simulink model "Cruise_Model_V16"  (R2024a)
settings: Solver=ode23t  StartTime=0.0  StopTime=t5(end)  RelTol=1e-3
values from neighbouring files (symbols this model uses):
  coefficients =     [UAM2.mat]    (also in VX4_cur.mat; VX4data.mat; alexisignoringme11UAM2.mat; alexisignoringme12.mat)
  idxf = [1 78 155 231 308 385 462 538 615 692 769 845 ... (70 elements, 1x70)]    [alexisignoringme.mat]    (also in alexisignoringme11UAM2.mat = [1 112 223 334 445 555 666 777 888 999 1001 1112 ... (50 ele; alexisignoringme12.mat = [1 54 106 159 211 264 316 369 421 474 526 579 ... (100 eleme; alexisignoringme13.mat = [1 54 106 159 211 264 316 369 421 474 526 579 ... (100 eleme; alexisignoringme14.mat = [1 500 999 1001 1500 1999 2001 2500 2999 3001 3500 3999 ... )
  Kpi = lqr(sys, Q, R)    [QRerr_LQI.m]    (also in alexisignoringme8.mat = [9.62344892608e-17 -1.21933000029e-16 1.4312558077e-15 29.45)
  missionruntime =     [alexisignoringme4.mat]    (also in alexisignoringme5.mat; alexisignoringme6.mat; alexisignoringme7.mat; alexisignoringme8.mat)
  q = 0.5*1.225*airflow.U^2    [VLMV3.m]    (also in VLMV3_modified.m = 0.5*1.225*airflow.U^2*Sref)
  Ut = [0 0 -4.89661324026e-08 0 0 -1504.57476188 -0.000428335964898 -1.57410795509e-09 3.42121377805e-06 0 0 0 ... (450 elements, 9x50)]    [alexisignoringme5.mat]    (also in alexisignoringme6.mat; alexisignoringme7.mat; alexisignoringme8.mat = [0 0 0 0 0 -1498.96331992 -4.41873387445e-05 -1.31180695462e)
  uvec = [0.1 3.42222222222 6.74444444444 10.0666666667 13.3888888889 16.7111111111 20.0333333333 23.3555555556 26.6777777778 30]    [alexisignoringme.mat]    (also in alexisignoringme4.mat; alexisignoringme5.mat; alexisignoringme6.mat; alexisignoringme7.mat)
  X = [0.00351660116596 0 -9.99999602467 0 0 0 2.75026701025e-08 -4.1982332666e-06 -1.5333765693e-08 0.000503097278932 0 -6.54626389426e-11 ... (630 elements, 9x5x14)]    [alexisignoringme.mat]    (also in alexisignoringme12.mat = [0.000256495736971 0 -9.99999647184 0 0 0 0 -3.73764411116e-; alexisignoringme13.mat = [0.00833666803911 0 -10.0000021435 0 0 0 0 7.14203458163e-06; alexisignoringme14.mat = [0.00833666803911 0 -10.0000021435 0 0 0 0 7.14203458163e-06; alexisignoringme4.mat = [0.00351658839646 0 -9.99999599468 0 0 0 2.7327442949e-09 -4)
  Xes = X(:,idx(4))    [QRerr_LQI.m]    (also in QRerr_p.m = X(:,idx(2)); alexisignoringme4.mat = [0.00351658839646 0 -9.99999599468 0 0 0 2.7327442949e-09 -4; alexisignoringme5.mat = [0 0 -1.11199998303 0 0 0 -1.38069247376e-09 1.48137256273e-; alexisignoringme6.mat = [0 0 -1.11199998303 0 0 0 -1.38069247376e-09 1.48137256273e-)
undefined symbols (not defined in the file or in its folder): F, Light, MIL, tl, VX4, xvec
libraries: slpidlib x14, aerolibwind2 x8, aerolibatmos2 x4, shared6dof x1
(part 2 of 3)

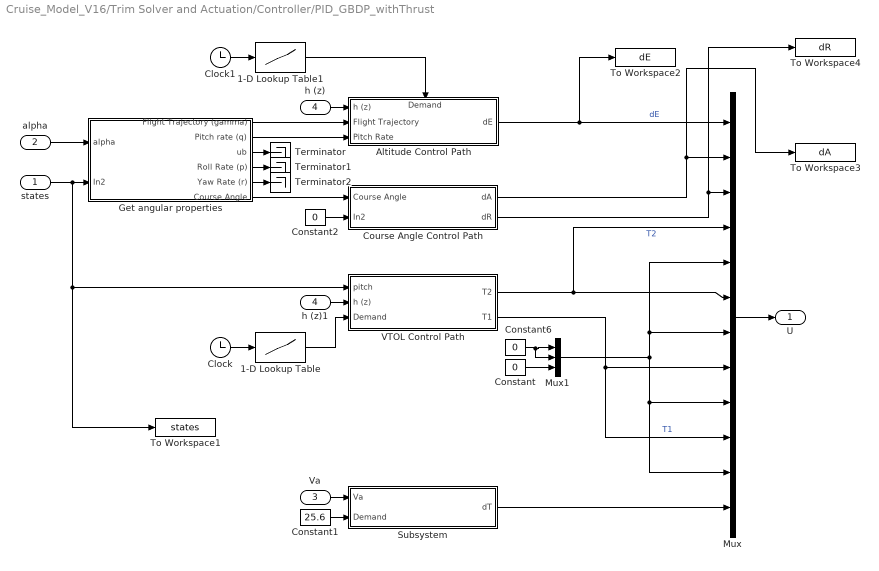
== system Cruise_Model_V16/Trim Solver and Actuation/Controller/PID_GBDP_withThrust ==
  states : Inport
  alpha : Inport  Port=2
  Va : Inport  Port=3
  h (z) : Inport  Port=4
  1-D Lookup Table : Lookup_n-D  NumberOfTableDimensions=1  BreakpointsForDimension1=[mission.trans.t mission.cruise.t(2:end)]  Table=[mission.trans.altitude 0*ones(size(mission.trans.altitude(2:end)))]  InternalRulePriority=Speed  RndMeth=Simplest
  1-D Lookup Table1 : Lookup_n-D  NumberOfTableDimensions=1  BreakpointsForDimension1=[mission.trans.t mission.cruise.t(2:end)]  Table=[mission.trans.altitude mission.cruise.altitude(2:end)]  InternalRulePriority=Speed  RndMeth=Simplest
  Altitude Control Path : Subsystem
      settings: PortSchema="{\"entries\":[{\"content\":{\"sides\":[{\"content\":{\"connectorIds\":[\"In1\",\"In2\",\"In3\"]},\"type\":\"ConnectorPlacement.EquallySpacedRectSide\",\"uuid\":\"675ebe7b-8fa8-41fa-ad50-d7fa74657396\"},{\"content\":{\"connectorIds\":[\"Out1\"],\"side\":\"RIGHT\"},\"type\":\"ConnectorPlacement.EquallySpacedRectSide\",\"uuid\":\"13b074cf-565d-449c-ab17-946bdb38993a\"},{\"content\":{\"connectorIds\":[\"In4\"],\"side\":\"TOP\"},\"type\":\"ConnectorPlacement.EquallySpacedRectSide\",\"uuid\":\"a25968b9-1287-4975-9ac3-b2da8f663380\"}]},\"type\":\"ConnectorPlacement.EquallySpacedConnector\",\"uuid\":\"28fe7750-cc88-4371-bcf6-f4778a62f5aa\"}],\"packageUris\":[\"http://schema.mathworks.com/mf0/Connector/R2020b\"],\"version\":\"1.0\"}"
  Clock : Clock
  Clock1 : Clock
  Constant : Constant  Value=0
  Constant1 : Constant  Value=25.6
  Constant2 : Constant  Value=0
  Constant6 : Constant  Value=0
  Course Angle Control Path : Subsystem
  Get angular properties : Subsystem
  Mux : Mux  Inputs=12
  Mux1 : Mux  Inputs=3
  Subsystem : Subsystem
  Terminator : Terminator
  Terminator1 : Terminator
  Terminator2 : Terminator
  To Workspace1 : ToWorkspace  VariableName=states  SaveFormat=Timeseries  SampleTime=-1
  To Workspace2 : ToWorkspace  VariableName=dE  SaveFormat=Timeseries  SampleTime=-1
  To Workspace3 : ToWorkspace  VariableName=dA  SaveFormat=Timeseries  SampleTime=-1
  To Workspace4 : ToWorkspace  VariableName=dR  SaveFormat=Timeseries  SampleTime=-1
  VTOL Control Path : Subsystem
  h (z)1 : InportShadow  Port=4
  U : Outport
  wires:
  Mux/1 -> U/1
  Get angular properties/5(Yaw Rate (r)) -> Terminator2/1
  Get angular properties/4(Roll Rate (p)) -> Terminator1/1
  alpha/1 -> Get angular properties/1(alpha)
  Get angular properties/3(ub) -> Terminator/1
  states/1 -> To Workspace1/1, VTOL Control Path/1(pitch), Get angular properties/2(In2)
  Mux1/1 -> Mux/5, Mux/7, Mux/11, Mux/9
  Constant6/1 -> Mux1/1, Mux1/2
  Constant/1 -> Mux1/3
  h (z)/1 -> Altitude Control Path/1(h (z))
  1-D Lookup Table1/1 -> Altitude Control Path/4(Demand)
  Get angular properties/1(Flight Trajectory (gamma)) -> Altitude Control Path/2(Flight Trajectory)
  Get angular properties/2(Pitch rate (q)) -> Altitude Control Path/3(Pitch Rate)
  Get angular properties/6(Course Angle) -> Course Angle Control Path/1(Course Angle)
  Va/1 -> Subsystem/1(Va)
  Constant1/1 -> Subsystem/2(Demand)
  Altitude Control Path/1(dE) -> Mux/1, To Workspace2/1  "dE"
  Course Angle Control Path/1(dA) -> To Workspace3/1, Mux/2
  Course Angle Control Path/2(dR) -> To Workspace4/1, Mux/3
  Clock/1 -> 1-D Lookup Table/1
  1-D Lookup Table/1 -> VTOL Control Path/3(Demand)
  h (z)1/1 -> VTOL Control Path/2(h (z))
  Clock1/1 -> 1-D Lookup Table1/1
  VTOL Control Path/1(T2) -> Mux/4, Mux/6  "T2"
  VTOL Control Path/2(T1) -> Mux/10, Mux/8  "T1"
  Subsystem/1(dT) -> Mux/12
  Constant2/1 -> Course Angle Control Path/2(In2)

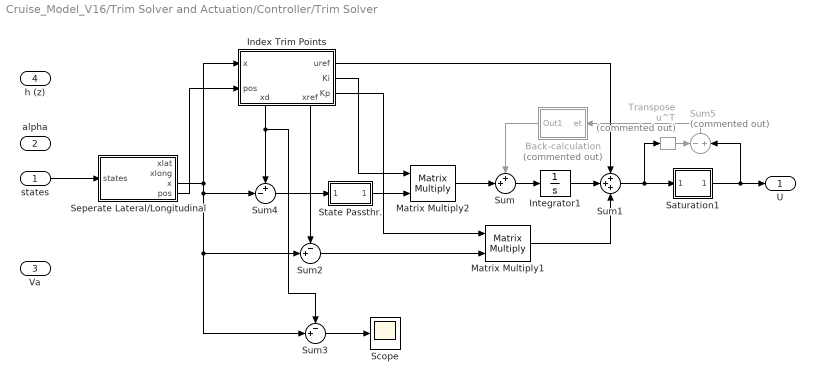
== system Cruise_Model_V16/Trim Solver and Actuation/Controller/Trim Solver ==
  states : Inport
  alpha : Inport  Port=2
  Va : Inport  Port=3
  h (z) : Inport  Port=4
  Back-calculation : Subsystem  Commented=on
  Index Trim Points : Subsystem
      settings: PortSchema="{\"entries\":[{\"content\":{\"sides\":[{\"content\":{\"connectorIds\":[\"In1\",\"In2\"]},\"type\":\"ConnectorPlacement.EquallySpacedRectSide\",\"uuid\":\"3e759be8-b0b5-4bdb-bb26-96e56af52772\"},{\"content\":{\"connectorIds\":[\"Out1\",\"Out2\",\"Out3\"],\"side\":\"RIGHT\"},\"type\":\"ConnectorPlacement.EquallySpacedRectSide\",\"uuid\":\"8308db73-24aa-4a70-a5f0-9ec5de8c120a\"},{\"content\":{\"side\":\"TOP\"},\"type\":\"ConnectorPlacement.EquallySpacedRectSide\",\"uuid\":\"2166a8af-7157-44fc-b4c0-6126f30836aa\"},{\"content\":{\"connectorIds\":[\"Out4\",\"Out5\"],\"side\":\"BOTTOM\"},\"type\":\"ConnectorPlacement.EquallySpacedRectSide\",\"uuid\":\"144aeecd-f2ed-4e8c-a5f9-9bd63c6f3635\"}]},\"type\":\"ConnectorPlacement.EquallySpacedConnector\",\"uuid\":\"70cf00ba-20c2-419b-abed-4793342c0662\"}],\"packageUris\":[\"http://schema.mathworks.com/mf0/Connector/R2020b\"],\"version\":\"1.0\"}"
  Integrator1 : Integrator
  Matrix Multiply1 : Product  Multiplication=Matrix(*)
  Matrix Multiply2 : Product  Multiplication=Matrix(*)
  Saturation1 : Subsystem
  Scope : Scope
  Seperate Lateral/Longitudinal : Subsystem
  State Passthr. : Subsystem
  Sum : Sum  Inputs=++|
  Sum1 : Sum  Inputs=+++
  Sum2 : Sum  Inputs=-+|
  Sum3 : Sum  Inputs=-+|
  Sum4 : Sum  Inputs=+-|
  Sum5 : Sum  Commented=on  Inputs=-|+
  Transpose : Math  Commented=on  Operator=transpose
  U : Outport
  wires:
  states/1 -> Seperate Lateral/Longitudinal/1(states)
  Index Trim Points/1(uref) -> Sum1/1
  Index Trim Points/4(xd) -> Sum3/1, Sum4/1
  Seperate Lateral/Longitudinal/3(x) -> Sum2/2, Sum3/2, Sum4/2, Index Trim Points/1(x)
  Index Trim Points/5(xref) -> Sum2/1
  Index Trim Points/3(Kp) -> Matrix Multiply1/1
  Index Trim Points/2(Ki) -> Matrix Multiply2/1
  Sum4/1 -> State Passthr./1(In2)
  State Passthr./1(Out4) -> Matrix Multiply2/2
  Sum2/1 -> Matrix Multiply1/2
  Sum1/1 -> Saturation1/1(In1), Transpose/1
  Matrix Multiply2/1 -> Sum/2
  Sum/1 -> Integrator1/1
  Transpose/1 -> Sum5/1
  Sum5/1 -> Back-calculation/1(et)
  Integrator1/1 -> Sum1/2
  Matrix Multiply1/1 -> Sum1/3
  Back-calculation/1(Out1) -> Sum/1
  Sum3/1 -> Scope/1
  Saturation1/1(Out1) -> Sum5/2, U/1
  Seperate Lateral/Longitudinal/4(pos) -> Index Trim Points/2(pos)

== system Cruise_Model_V16/Atmospheric Effects/Atmospheric Effects1/Variant Subsystem/a ==
  h (z) : Inport
  Constant : Constant  Value=0
  ISA Atmosphere : aerolibatmos2/ISA Atmosphere Model  useExtended=off  action=Warning  custom=off  viscosityOut=off  g=9.80665  gamma=1.4  R=287.0531  L=0.0065  h_trop=11000  h_strat=20000  rho0=1.225  P0=101325  T0=288.15  h0=0  S=110.4  Tref=273.15  muref=1.716e-5
  Terminator1 : Terminator
  Terminator2 : Terminator
  Terminator3 : Terminator
  Air Density : Outport
  Vw : Outport  Port=2
  wires:
  h (z)/1 -> ISA Atmosphere/1
  ISA Atmosphere/2 -> Terminator1/1
  ISA Atmosphere/1 -> Terminator3/1
  ISA Atmosphere/4 -> Air Density/1
  ISA Atmosphere/3 -> Terminator2/1
  Constant/1 -> Vw/1

== system Cruise_Model_V16/Atmospheric Effects/Atmospheric Effects1/Variant Subsystem/ag ==
  uvw_e : Inport
  h (z) : Inport  Port=2
  Demux : Demux  Outputs=3
  Discrete Wind Gust Model : aerolibwind2/Discrete Wind Gust Model  units=Metric (MKS)  Gx=on  Gy=on  Gz=on  t_0=40  d_m=[120 120 80]  v_m=[10 10 10]
  ISA Atmosphere : aerolibatmos2/ISA Atmosphere Model  custom=off  g=9.80665  gamma=1.4  R=287.0531  L=0.0065  h_trop=11000  h_strat=20000  rho0=1.225  P0=101325  T0=288.15  h0=0
  Terminator1 : Terminator
  Terminator2 : Terminator
  Terminator3 : Terminator
  Vw : Outport
  Air Density : Outport  Port=2
  wires:
  h (z)/1 -> ISA Atmosphere/1
  Demux/1 -> Discrete Wind Gust Model/1
  ISA Atmosphere/2 -> Terminator1/1
  ISA Atmosphere/1 -> Terminator3/1
  ISA Atmosphere/4 -> Air Density/1
  uvw_e/1 -> Demux/1
  ISA Atmosphere/3 -> Terminator2/1
  Discrete Wind Gust Model/1 -> Vw/1

== system Cruise_Model_V16/Atmospheric Effects/Atmospheric Effects1/Variant Subsystem/agt ==
  <uvw_e> : Inport
  DCM : Inport  Port=2
  h (z) : Inport  Port=3
  Demux : Demux  Outputs=3
  Discrete Wind Gust Model : aerolibwind2/Discrete Wind Gust Model  units=Metric (MKS)  Gx=on  Gy=on  Gz=on  t_0=40  d_m=[120 120 80]  v_m=[10 10 10]
  Dryden Wind Turbulence Model (Discrete (+q +r)) : aerolibwind2/Dryden Wind Turbulence Model  (Continuous (+q -r))  units=Metric (MKS)  spec=MIL-F-8785C  model=Continuous Dryden (+q -r)  W20=10  Wdeg=8  TurbProb=10^-2 - Light  L_high=533.4  Wingspan=7  ts=0.1  Seed=[23341 23342 23343 23344]  T_on=on
      settings: LibrarySourceBlock=|
      | aerolibwind2/Dryden Wind Turbulence Model
      | (Discrete (+q +r))
  ISA Atmosphere : aerolibatmos2/ISA Atmosphere Model  custom=off  g=9.80665  gamma=1.4  R=287.0531  L=0.0065  h_trop=11000  h_strat=20000  rho0=1.225  P0=101325  T0=288.15  h0=0
  Sum : Sum  Inputs=|++
  Terminator{,1..3} (4 alike) : Terminator
  Vw : Outport
  Air Density : Outport  Port=2
  wires:
  h (z)/1 -> Dryden Wind Turbulence Model (Discrete (+q +r))/1, ISA Atmosphere/1
  Demux/1 -> Dryden Wind Turbulence Model (Discrete (+q +r))/2, Discrete Wind Gust Model/1
  ISA Atmosphere/2 -> Terminator1/1
  ISA Atmosphere/1 -> Terminator3/1
  ISA Atmosphere/4 -> Air Density/1
  <uvw_e>/1 -> Demux/1
  DCM/1 -> Dryden Wind Turbulence Model (Discrete (+q +r))/3
  Dryden Wind Turbulence Model (Discrete (+q +r))/2 -> Terminator/1
  Sum/1 -> Vw/1
  ISA Atmosphere/3 -> Terminator2/1
  Dryden Wind Turbulence Model (Discrete (+q +r))/1 -> Sum/2
  Discrete Wind Gust Model/1 -> Sum/1

== system Cruise_Model_V16/Atmospheric Effects/Atmospheric Effects1/Variant Subsystem/at ==
  uvw_e : Inport
  DCM : Inport  Port=2
  h (z) : Inport  Port=3
  Demux : Demux  Outputs=3
  Dryden Wind Turbulence Model (Discrete (+q +r)) : aerolibwind2/Dryden Wind Turbulence Model  (Continuous (+q -r))  units=Metric (MKS)  spec=MIL-F-8785C  model=Continuous Dryden (+q -r)  W20=10  Wdeg=8  TurbProb=10^-2 - Light  L_high=533.4  Wingspan=7  ts=0.1  Seed=[23341 23342 23343 23344]  T_on=on
      settings: LibrarySourceBlock=|
      | aerolibwind2/Dryden Wind Turbulence Model
      | (Discrete (+q +r))
  ISA Atmosphere : aerolibatmos2/ISA Atmosphere Model  custom=off  g=9.80665  gamma=1.4  R=287.0531  L=0.0065  h_trop=11000  h_strat=20000  rho0=1.225  P0=101325  T0=288.15  h0=0
  Terminator{,1..5} (6 alike) : Terminator
  Vw : Outport
  Air Density : Outport  Port=2
  wires:
  h (z)/1 -> Dryden Wind Turbulence Model (Discrete (+q +r))/1, ISA Atmosphere/1
  Demux/1 -> Dryden Wind Turbulence Model (Discrete (+q +r))/2
  ISA Atmosphere/2 -> Terminator1/1
  ISA Atmosphere/1 -> Terminator3/1
  ISA Atmosphere/4 -> Air Density/1
  uvw_e/1 -> Demux/1
  DCM/1 -> Dryden Wind Turbulence Model (Discrete (+q +r))/3
  Dryden Wind Turbulence Model (Discrete (+q +r))/2 -> Terminator/1
  ISA Atmosphere/3 -> Terminator2/1
  Demux/2 -> Terminator4/1
  Demux/3 -> Terminator5/1
  Dryden Wind Turbulence Model (Discrete (+q +r))/1 -> Vw/1

== system Cruise_Model_V16/Atmospheric Effects/Atmospheric Effects1/Variant Subsystem/g ==
  uvw_e : Inport
  Constant : Constant  Value=1.225
  Demux : Demux  Outputs=3
  Discrete Wind Gust Model : aerolibwind2/Discrete Wind Gust Model  units=Metric (MKS)  Gx=on  Gy=on  Gz=on  t_0=40  d_m=[120 120 80]  v_m=[10 10 10]
  Vw : Outport
  Air Density : Outport  Port=2
  wires:
  Demux/1 -> Discrete Wind Gust Model/1
  uvw_e/1 -> Demux/1
  Discrete Wind Gust Model/1 -> Vw/1
  Constant/1 -> Air Density/1

== system Cruise_Model_V16/Atmospheric Effects/Atmospheric Effects1/Variant Subsystem/gt ==
  <uvw_e> : Inport
  DCM : Inport  Port=2
  h (z) : Inport  Port=3
  Constant : Constant  Value=1.225
  Demux : Demux  Outputs=3
  Discrete Wind Gust Model : aerolibwind2/Discrete Wind Gust Model  units=Metric (MKS)  Gx=on  Gy=on  Gz=on  t_0=40  d_m=[120 120 80]  v_m=[10 10 10]
  Dryden Wind Turbulence Model (Discrete (+q +r)) : aerolibwind2/Dryden Wind Turbulence Model  (Continuous (+q -r))  units=Metric (MKS)  spec=MIL-F-8785C  model=Continuous Dryden (+q -r)  W20=10  Wdeg=8  TurbProb=10^-2 - Light  L_high=533.4  Wingspan=7  ts=0.1  Seed=[23341 23342 23343 23344]  T_on=on
      settings: LibrarySourceBlock=|
      | aerolibwind2/Dryden Wind Turbulence Model
      | (Discrete (+q +r))
  Sum : Sum  Inputs=|++
  Terminator : Terminator
  Vw : Outport
  Air Density : Outport  Port=2
  wires:
  h (z)/1 -> Dryden Wind Turbulence Model (Discrete (+q +r))/1
  Demux/1 -> Dryden Wind Turbulence Model (Discrete (+q +r))/2, Discrete Wind Gust Model/1
  <uvw_e>/1 -> Demux/1
  DCM/1 -> Dryden Wind Turbulence Model (Discrete (+q +r))/3
  Dryden Wind Turbulence Model (Discrete (+q +r))/2 -> Terminator/1
  Sum/1 -> Vw/1
  Dryden Wind Turbulence Model (Discrete (+q +r))/1 -> Sum/2
  Discrete Wind Gust Model/1 -> Sum/1
  Constant/1 -> Air Density/1

== system Cruise_Model_V16/Atmospheric Effects/Atmospheric Effects1/Variant Subsystem/n ==
  Constant : Constant  Value=0
  Constant1 : Constant  Value=1.225
  Vw : Outport
  Air Density : Outport  Port=2
  wires:
  Constant/1 -> Vw/1
  Constant1/1 -> Air Density/1

== system Cruise_Model_V16/Atmospheric Effects/Atmospheric Effects1/Variant Subsystem/t ==
  <uvw_e> : Inport
  DCM : Inport  Port=2
  h (z) : Inport  Port=3
  Constant1 : Constant  Value=1.225
  Demux : Demux  Outputs=3
  Dryden Wind Turbulence Model (Discrete (+q +r)) : aerolibwind2/Dryden Wind Turbulence Model  (Continuous (+q -r))  units=Metric (MKS)  spec=MIL-F-8785C  model=Continuous Dryden (+q -r)  W20=10  Wdeg=8  TurbProb=10^-2 - Light  L_high=533.4  Wingspan=7  ts=0.1  Seed=[23341 23342 23343 23344]  T_on=on
      settings: LibrarySourceBlock=|
      | aerolibwind2/Dryden Wind Turbulence Model
      | (Discrete (+q +r))
  Terminator : Terminator
  Vw : Outport
  Air Density : Outport  Port=2
  wires:
  h (z)/1 -> Dryden Wind Turbulence Model (Discrete (+q +r))/1
  Demux/1 -> Dryden Wind Turbulence Model (Discrete (+q +r))/2
  <uvw_e>/1 -> Demux/1
  DCM/1 -> Dryden Wind Turbulence Model (Discrete (+q +r))/3
  Dryden Wind Turbulence Model (Discrete (+q +r))/2 -> Terminator/1
  Constant1/1 -> Air Density/1
  Dryden Wind Turbulence Model (Discrete (+q +r))/1 -> Vw/1

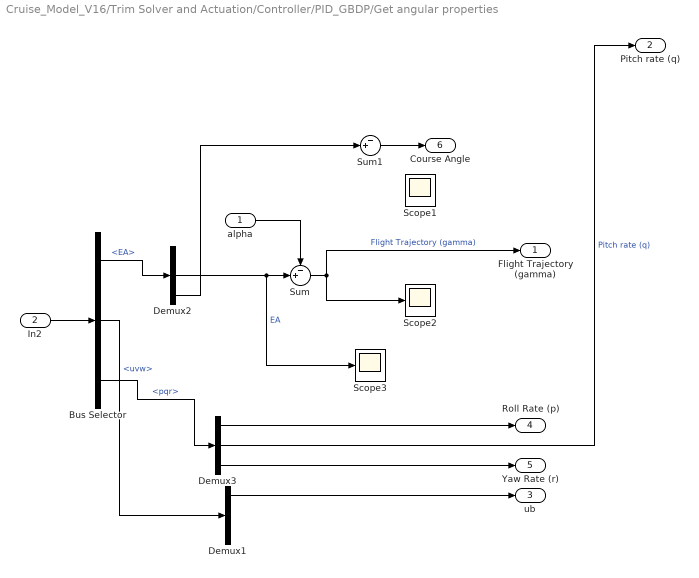
== system Cruise_Model_V16/Trim Solver and Actuation/Controller/PID_GBDP/Get angular properties ==
  alpha : Inport
  In2 : Inport  Port=2
  Bus Selector : BusSelector  OutputSignals=EA,uvw,pqr
  Demux1 : Demux  Outputs=3
  Demux2 : Demux  Outputs=3
  Demux3 : Demux  Outputs=3
  Scope1 : Scope
  Scope2 : Scope
  Scope3 : Scope
  Sum : Sum  Inputs=-+|
  Sum1 : Sum  Inputs=-+|
  Flight Trajectory (gamma) : Outport
  Pitch rate (q) : Outport  Port=2
  ub : Outport  Port=3
  Roll Rate (p) : Outport  Port=4
  Yaw Rate (r) : Outport  Port=5
  Course Angle : Outport  Port=6
  wires:
  alpha/1 -> Sum/1
  Demux2/2 -> Sum/2, Scope3/1  "EA"
  Bus Selector/3 -> Demux3/1  "<pqr>"
  Sum/1 -> Flight Trajectory (gamma)/1, Scope2/1  "Flight Trajectory (gamma)"
  Bus Selector/1 -> Demux2/1  "<EA>"
  In2/1 -> Bus Selector/1
  Demux3/2 -> Pitch rate (q)/1  "Pitch rate (q)"
  Bus Selector/2 -> Demux1/1  "<uvw>"
  Demux1/1 -> ub/1
  Demux3/1 -> Roll Rate (p)/1
  Sum1/1 -> Course Angle/1
  Demux3/3 -> Yaw Rate (r)/1
  Demux2/3 -> Sum1/2

== system Cruise_Model_V16/Trim Solver and Actuation/Controller/PID_GBDP/Step demand for testing ==
  In1 : Inport
  Mux1 : Mux  Inputs=2
  Scope2 : Scope
  Scope4 : Scope
  Step1 : Step  Time=60  Before=-500  After=-490  SampleTime=0
  Step2 : Step  Time=80  After=-10  SampleTime=0
  Step3 : Step  Time=120  After=20  SampleTime=0
  Step4 : Step  Time=120  After=20  SampleTime=0
  Sum : Sum  Inputs=++++
  To Workspace : ToWorkspace  VariableName=altitudeResponse  SaveFormat=Timeseries  SampleTime=-1
  Out1 : Outport
  wires:
  Step3/1 -> Sum/3
  Mux1/1 -> To Workspace/1, Scope4/1
  Sum/1 -> Out1/1, Mux1/1
  Step4/1 -> Sum/4
  Step1/1 -> Sum/1
  In1/1 -> Mux1/2, Scope2/1
  Step2/1 -> Sum/2

== system Cruise_Model_V16/Trim Solver and Actuation/Controller/PID_GBDP/Step demand for testing1 ==
  Va : Inport
  Mux1 : Mux  Inputs=2
  Scope2 : Scope
  Scope4 : Scope
  Step1 : Step  Time=60  Before=25  After=31  SampleTime=0
  Step2 : Step  Time=80  After=-3  SampleTime=0
  Step3 : Step  Time=120  After=-5  SampleTime=0
  Step4 : Step  Time=100  After=8  SampleTime=0
  Step5 : Step  Time=140  After=-2  SampleTime=0
  Sum : Sum  Inputs=+++++
  To Workspace : ToWorkspace  VariableName=airspeedResponse  SaveFormat=Timeseries  SampleTime=-1
  Out1 : Outport
  wires:
  Step2/1 -> Sum/2
  Va/1 -> Scope2/1, Mux1/2
  Step1/1 -> Sum/1
  Step4/1 -> Sum/4
  Sum/1 -> Mux1/1, Out1/1
  Mux1/1 -> Scope4/1, To Workspace/1
  Step3/1 -> Sum/3
  Step5/1 -> Sum/5

== system Cruise_Model_V16/Trim Solver and Actuation/Controller/PID_GBDP/Step demand for testing2 ==
  Va : Inport
  Mux1 : Mux  Inputs=2
  Scope2 : Scope
  Scope4 : Scope
  Step1 : Step  Time=60  Before=0.1  After=0.2  SampleTime=0
  Step2 : Step  Time=80  After=-0.4  SampleTime=0
  Step3 : Step  Time=120  After=-0.2  SampleTime=0
  Step4 : Step  Time=100  After=0.6  SampleTime=0
  Step5 : Step  Time=140  After=-0.4  SampleTime=0
  Sum : Sum  Inputs=+++++
  To Workspace : ToWorkspace  VariableName=headingAngleResponse  SaveFormat=Timeseries  SampleTime=-1
  Out1 : Outport
  wires:
  Step5/1 -> Sum/5
  Step3/1 -> Sum/3
  Mux1/1 -> To Workspace/1, Scope4/1
  Sum/1 -> Out1/1, Mux1/1
  Step4/1 -> Sum/4
  Step1/1 -> Sum/1
  Va/1 -> Mux1/2, Scope2/1
  Step2/1 -> Sum/2

== system Cruise_Model_V16/Trim Solver and Actuation/Controller/PID_GBDP_withThrust/Altitude Control Path ==
  note: Altitude Control Path
  h (z) : Inport
  Flight Trajectory : Inport  Port=2
  Pitch Rate : Inport  Port=3
  Demand : Inport  Port=4
  PID Controller10 : slpidlib/PID Controller  Controller=PID  Form=Parallel  TimeDomain=Continuous-time  UseExternalTs=off  SampleTime=-1  IntegratorMethod=Forward Euler  FilterMethod=Forward Euler  ControllerParametersSource=internal  P=-0.89713711901533  I=-27.659938076894  UseKiTs=off  D=-0.00302643608728309  N=142.832860389355  UseFilter=on  TunerSelectOption=Transfer Function Based (PID Tuner App)  InitialConditionSource=internal  InitialConditionForIntegrator=0.44  InitialConditionForFilter=0  DifferentiatorICPrevScaledInput=0  ExternalReset=none  TrackingMode=off  Kt=1  LimitOutput=on  SatLimitsSource=internal  UpperSaturationLimit=0.44  LowerSaturationLimit=-0.44  LinearizeAsGain=on  AntiWindupMode=clamping  Kb=1  LimitIntegrator=off  UpperIntegratorSaturationLimit=inf  LowerIntegratorSaturationLimit=-inf  POutMin=[]  POutMax=[]  IOutMin=[]  IOutMax=[]  DOutMin=[]  DOutMax=[]  NOutMin=[]  NOutMax=[]  SumOutMin=[]  SumOutMax=[]  SaturationOutMin=[]  SaturationOutMax=[]  PParamMin=[]  PParamMax=[]  IParamMin=[]  IParamMax=[]  DParamMin=[]  DParamMax=[]  NParamMin=[]  NParamMax=[]  KbParamMin=[]  KbParamMax=[]  KtParamMin=[]  KtParamMax=[]  KbOutMin=[]  KbOutMax=[]  KtOutMin=[]  KtOutMax=[]  IntegratorOutMin=[]  IntegratorOutMax=[]  FilterOutMin=[]  FilterOutMax=[]  SumI1OutMin=[]  SumI1OutMax=[]  SumI2OutMin=[]  SumI2OutMax=[]  SumI3OutMin=[]  SumI3OutMax=[]  SumI4OutMin=[]  SumI4OutMax=[]  SumDOutMin=[]  SumDOutMax=[]  DifferentiatorOutMin=[]  DifferentiatorOutMax=[]  FilterDiffOutCoefMin=[]  FilterDiffOutCoefMax=[]  ReciprocalOutMin=[]  ReciprocalOutMax=[]  SumDenOutMin=[]  SumDenOutMax=[]  SumNumOutMin=[]  SumNumOutMax=[]  DivideOutMin=[]  DivideOutMax=[]  UdiffTsProdOutMin=[]  UdiffTsProdOutMax=[]  NTsProdOutMin=[]  NTsProdOutMax=[]  UintegralTsProdOutMin=[]  UintegralTsProdOutMax=[]  UngainTsProdOutMin=[]  UngainTsProdOutMax=[]  ClampingZeroOutDataTypeStr=Inherit: Inherit via back propagation  ClampingZeroOutMin=[]  ClampingZeroOutMax=[]  FilterDenConstantOutDataTypeStr=Inherit: Inherit via back propagation  FilterDenConstantOutMin=[]  FilterDenConstantOutMax=[]  PCopyOutDataTypeStr=Inherit: Inherit via back propagation  PCopyOutMin=[]  PCopyOutMax=[]  NCopyOutDataTypeStr=Inherit: Inherit via back propagation  NCopyOutMin=[]  NCopyOutMax=[]  IntegratorContinuousStateAttributes=''  IntegratorStateMustResolveToSignalObject=off  IntegratorRTWStateStorageClass=Auto  FilterContinuousStateAttributes=''  FilterStateMustResolveToSignalObject=off  FilterRTWStateStorageClass=Auto  ParallelPVariant=InternalParameters  IdealPVariant=Disabled  IVariant=InternalParameters  DVariant=InternalParameters  IntegratorVariant=Continuous  SatVariant=Enabled  AWVariant=ContClampingParallel  PCopyVariant=Disabled  TRVariant=Disabled  FdbkBlocksVariant=Forward  IdealPFdbkVariant=Disabled  SatFdbkVariant=Disabled  DerivativeFilterVariant=ContFilter  NVariant=InternalParameters  NCopyVariant=Disabled  FilterICVariant=InternalICsFilter  IntegratorICVariant=InternalICs  ExternalResetVariant=Disabled  TRSumVariant=Passthrough  SumFdbkVariant=Disabled  SumVariant=Sum_PID  TsampFilterVariant=InternalTs  TsampNgainVariant=Passthrough  TsampIntegralVariant=Passthrough  ExternalSaturationOutDataTypeStr=Inherit: Same as second input
  PID Controller4 : slpidlib/PID Controller  Controller=PID  Form=Parallel  TimeDomain=Continuous-time  UseExternalTs=off  SampleTime=-1  IntegratorMethod=Forward Euler  FilterMethod=Forward Euler  ControllerParametersSource=internal  P=-0.487630187489664  I=-0.0704619791070383  UseKiTs=off  D=-0.813392530162756  N=7.99704030727873  UseFilter=on  TunerSelectOption=Transfer Function Based (PID Tuner App)  InitialConditionSource=internal  InitialConditionForIntegrator=0.1  InitialConditionForFilter=0  DifferentiatorICPrevScaledInput=0  ExternalReset=none  TrackingMode=off  Kt=1  LimitOutput=on  SatLimitsSource=internal  UpperSaturationLimit=0.44  LowerSaturationLimit=-0.44  LinearizeAsGain=on  AntiWindupMode=clamping  Kb=1  LimitIntegrator=off  UpperIntegratorSaturationLimit=inf  LowerIntegratorSaturationLimit=-inf  POutMin=[]  POutMax=[]  IOutMin=[]  IOutMax=[]  DOutMin=[]  DOutMax=[]  NOutMin=[]  NOutMax=[]  SumOutMin=[]  SumOutMax=[]  SaturationOutMin=[]  SaturationOutMax=[]  PParamMin=[]  PParamMax=[]  IParamMin=[]  IParamMax=[]  DParamMin=[]  DParamMax=[]  NParamMin=[]  NParamMax=[]  KbParamMin=[]  KbParamMax=[]  KtParamMin=[]  KtParamMax=[]  KbOutMin=[]  KbOutMax=[]  KtOutMin=[]  KtOutMax=[]  IntegratorOutMin=[]  IntegratorOutMax=[]  FilterOutMin=[]  FilterOutMax=[]  SumI1OutMin=[]  SumI1OutMax=[]  SumI2OutMin=[]  SumI2OutMax=[]  SumI3OutMin=[]  SumI3OutMax=[]  SumI4OutMin=[]  SumI4OutMax=[]  SumDOutMin=[]  SumDOutMax=[]  DifferentiatorOutMin=[]  DifferentiatorOutMax=[]  FilterDiffOutCoefMin=[]  FilterDiffOutCoefMax=[]  ReciprocalOutMin=[]  ReciprocalOutMax=[]  SumDenOutMin=[]  SumDenOutMax=[]  SumNumOutMin=[]  SumNumOutMax=[]  DivideOutMin=[]  DivideOutMax=[]  UdiffTsProdOutMin=[]  UdiffTsProdOutMax=[]  NTsProdOutMin=[]  NTsProdOutMax=[]  UintegralTsProdOutMin=[]  UintegralTsProdOutMax=[]  UngainTsProdOutMin=[]  UngainTsProdOutMax=[]  ClampingZeroOutDataTypeStr=Inherit: Inherit via back propagation  ClampingZeroOutMin=[]  ClampingZeroOutMax=[]  FilterDenConstantOutDataTypeStr=Inherit: Inherit via back propagation  FilterDenConstantOutMin=[]  FilterDenConstantOutMax=[]  PCopyOutDataTypeStr=Inherit: Inherit via back propagation  PCopyOutMin=[]  PCopyOutMax=[]  NCopyOutDataTypeStr=Inherit: Inherit via back propagation  NCopyOutMin=[]  NCopyOutMax=[]  IntegratorContinuousStateAttributes=''  IntegratorStateMustResolveToSignalObject=off  IntegratorRTWStateStorageClass=Auto  FilterContinuousStateAttributes=''  FilterStateMustResolveToSignalObject=off  FilterRTWStateStorageClass=Auto  ParallelPVariant=InternalParameters  IdealPVariant=Disabled  IVariant=InternalParameters  DVariant=InternalParameters  IntegratorVariant=Continuous  SatVariant=Enabled  AWVariant=ContClampingParallel  PCopyVariant=Disabled  TRVariant=Disabled  FdbkBlocksVariant=Forward  IdealPFdbkVariant=Disabled  SatFdbkVariant=Disabled  DerivativeFilterVariant=ContFilter  NVariant=InternalParameters  NCopyVariant=Disabled  FilterICVariant=InternalICsFilter  IntegratorICVariant=InternalICs  ExternalResetVariant=Disabled  TRSumVariant=Passthrough  SumFdbkVariant=Disabled  SumVariant=Sum_PID  TsampFilterVariant=InternalTs  TsampNgainVariant=Passthrough  TsampIntegralVariant=Passthrough  ExternalSaturationOutDataTypeStr=Inherit: Same as second input
  PID Controller9 : slpidlib/PID Controller  Controller=PID  Form=Parallel  TimeDomain=Continuous-time  UseExternalTs=off  SampleTime=-1  IntegratorMethod=Forward Euler  FilterMethod=Forward Euler  ControllerParametersSource=internal  P=0.0886412010406481  I=0.0145723289748373  UseKiTs=off  D=0.129850691124493  N=8.9831666478447  UseFilter=on  TunerSelectOption=Transfer Function Based (PID Tuner App)  InitialConditionSource=internal  InitialConditionForIntegrator=0  InitialConditionForFilter=0  DifferentiatorICPrevScaledInput=0  ExternalReset=none  TrackingMode=off  Kt=1  LimitOutput=on  SatLimitsSource=internal  UpperSaturationLimit=0.09  LowerSaturationLimit=-0.3  LinearizeAsGain=off  AntiWindupMode=clamping  Kb=1  LimitIntegrator=off  UpperIntegratorSaturationLimit=inf  LowerIntegratorSaturationLimit=-inf  POutMin=[]  POutMax=[]  IOutMin=[]  IOutMax=[]  DOutMin=[]  DOutMax=[]  NOutMin=[]  NOutMax=[]  SumOutMin=[]  SumOutMax=[]  SaturationOutMin=[]  SaturationOutMax=[]  PParamMin=[]  PParamMax=[]  IParamMin=[]  IParamMax=[]  DParamMin=[]  DParamMax=[]  NParamMin=[]  NParamMax=[]  KbParamMin=[]  KbParamMax=[]  KtParamMin=[]  KtParamMax=[]  KbOutMin=[]  KbOutMax=[]  KtOutMin=[]  KtOutMax=[]  IntegratorOutMin=[]  IntegratorOutMax=[]  FilterOutMin=[]  FilterOutMax=[]  SumI1OutMin=[]  SumI1OutMax=[]  SumI2OutMin=[]  SumI2OutMax=[]  SumI3OutMin=[]  SumI3OutMax=[]  SumI4OutMin=[]  SumI4OutMax=[]  SumDOutMin=[]  SumDOutMax=[]  DifferentiatorOutMin=[]  DifferentiatorOutMax=[]  FilterDiffOutCoefMin=[]  FilterDiffOutCoefMax=[]  ReciprocalOutMin=[]  ReciprocalOutMax=[]  SumDenOutMin=[]  SumDenOutMax=[]  SumNumOutMin=[]  SumNumOutMax=[]  DivideOutMin=[]  DivideOutMax=[]  UdiffTsProdOutMin=[]  UdiffTsProdOutMax=[]  NTsProdOutMin=[]  NTsProdOutMax=[]  UintegralTsProdOutMin=[]  UintegralTsProdOutMax=[]  UngainTsProdOutMin=[]  UngainTsProdOutMax=[]  ClampingZeroOutDataTypeStr=Inherit: Inherit via back propagation  ClampingZeroOutMin=[]  ClampingZeroOutMax=[]  FilterDenConstantOutDataTypeStr=Inherit: Inherit via back propagation  FilterDenConstantOutMin=[]  FilterDenConstantOutMax=[]  PCopyOutDataTypeStr=Inherit: Inherit via back propagation  PCopyOutMin=[]  PCopyOutMax=[]  NCopyOutDataTypeStr=Inherit: Inherit via back propagation  NCopyOutMin=[]  NCopyOutMax=[]  IntegratorContinuousStateAttributes=''  IntegratorStateMustResolveToSignalObject=off  IntegratorRTWStateStorageClass=Auto  FilterContinuousStateAttributes=''  FilterStateMustResolveToSignalObject=off  FilterRTWStateStorageClass=Auto  ParallelPVariant=InternalParameters  IdealPVariant=Disabled  IVariant=InternalParameters  DVariant=InternalParameters  IntegratorVariant=Continuous  SatVariant=Enabled  AWVariant=ContClampingParallel  PCopyVariant=Disabled  TRVariant=Disabled  FdbkBlocksVariant=Forward  IdealPFdbkVariant=Disabled  SatFdbkVariant=Disabled  DerivativeFilterVariant=ContFilter  NVariant=InternalParameters  NCopyVariant=Disabled  FilterICVariant=InternalICsFilter  IntegratorICVariant=InternalICs  ExternalResetVariant=Disabled  TRSumVariant=Passthrough  SumFdbkVariant=Disabled  SumVariant=Sum_PID  TsampFilterVariant=InternalTs  TsampNgainVariant=Passthrough  TsampIntegralVariant=Passthrough  ExternalSaturationOutDataTypeStr=Inherit: Same as second input
  Step demand for testing : Subsystem
  Subtract : Sum  Inputs=|-+
  Subtract1 : Sum  Inputs=|+-
  Subtract3 : Sum  Inputs=|-+
  dE : Outport
  wires:
  PID Controller9/1 -> Subtract/1
  h (z)/1 -> Step demand for testing/1(In1), Subtract1/1
  Subtract/1 -> PID Controller4/1
  Pitch Rate/1 -> Subtract3/2
  Subtract1/1 -> PID Controller9/1
  Subtract3/1 -> PID Controller10/1
  PID Controller4/1 -> Subtract3/1
  Flight Trajectory/1 -> Subtract/2
  PID Controller10/1 -> dE/1
  Demand/1 -> Subtract1/2

== system Cruise_Model_V16/Trim Solver and Actuation/Controller/PID_GBDP_withThrust/Course Angle Control Path ==
  note: Course Angle Control Path
  Course Angle : Inport
  In2 : Inport  Port=2
  PID Controller2 : slpidlib/PID Controller  Controller=PID  Form=Parallel  TimeDomain=Continuous-time  UseExternalTs=off  SampleTime=-1  IntegratorMethod=Forward Euler  FilterMethod=Forward Euler  ControllerParametersSource=internal  P=0.61259661356046  I=0.000997427544306601  UseKiTs=off  D=0.894500555152138  N=62.5354170285902  UseFilter=on  TunerSelectOption=Transfer Function Based (PID Tuner App)  InitialConditionSource=internal  InitialConditionForIntegrator=0  InitialConditionForFilter=0  DifferentiatorICPrevScaledInput=0  ExternalReset=none  TrackingMode=off  Kt=1  LimitOutput=on  SatLimitsSource=internal  UpperSaturationLimit=0.52  LowerSaturationLimit=-0.52  LinearizeAsGain=on  AntiWindupMode=clamping  Kb=1  LimitIntegrator=off  UpperIntegratorSaturationLimit=inf  LowerIntegratorSaturationLimit=-inf  POutMin=[]  POutMax=[]  IOutMin=[]  IOutMax=[]  DOutMin=[]  DOutMax=[]  NOutMin=[]  NOutMax=[]  SumOutMin=[]  SumOutMax=[]  SaturationOutMin=[]  SaturationOutMax=[]  PParamMin=[]  PParamMax=[]  IParamMin=[]  IParamMax=[]  DParamMin=[]  DParamMax=[]  NParamMin=[]  NParamMax=[]  KbParamMin=[]  KbParamMax=[]  KtParamMin=[]  KtParamMax=[]  KbOutMin=[]  KbOutMax=[]  KtOutMin=[]  KtOutMax=[]  IntegratorOutMin=[]  IntegratorOutMax=[]  FilterOutMin=[]  FilterOutMax=[]  SumI1OutMin=[]  SumI1OutMax=[]  SumI2OutMin=[]  SumI2OutMax=[]  SumI3OutMin=[]  SumI3OutMax=[]  SumI4OutMin=[]  SumI4OutMax=[]  SumDOutMin=[]  SumDOutMax=[]  DifferentiatorOutMin=[]  DifferentiatorOutMax=[]  FilterDiffOutCoefMin=[]  FilterDiffOutCoefMax=[]  ReciprocalOutMin=[]  ReciprocalOutMax=[]  SumDenOutMin=[]  SumDenOutMax=[]  SumNumOutMin=[]  SumNumOutMax=[]  DivideOutMin=[]  DivideOutMax=[]  UdiffTsProdOutMin=[]  UdiffTsProdOutMax=[]  NTsProdOutMin=[]  NTsProdOutMax=[]  UintegralTsProdOutMin=[]  UintegralTsProdOutMax=[]  UngainTsProdOutMin=[]  UngainTsProdOutMax=[]  ClampingZeroOutDataTypeStr=Inherit: Inherit via back propagation  ClampingZeroOutMin=[]  ClampingZeroOutMax=[]  FilterDenConstantOutDataTypeStr=Inherit: Inherit via back propagation  FilterDenConstantOutMin=[]  FilterDenConstantOutMax=[]  PCopyOutDataTypeStr=Inherit: Inherit via back propagation  PCopyOutMin=[]  PCopyOutMax=[]  NCopyOutDataTypeStr=Inherit: Inherit via back propagation  NCopyOutMin=[]  NCopyOutMax=[]  IntegratorContinuousStateAttributes=''  IntegratorStateMustResolveToSignalObject=off  IntegratorRTWStateStorageClass=Auto  FilterContinuousStateAttributes=''  FilterStateMustResolveToSignalObject=off  FilterRTWStateStorageClass=Auto  ParallelPVariant=InternalParameters  IdealPVariant=Disabled  IVariant=InternalParameters  DVariant=InternalParameters  IntegratorVariant=Continuous  SatVariant=Enabled  AWVariant=ContClampingParallel  PCopyVariant=Disabled  TRVariant=Disabled  FdbkBlocksVariant=Forward  IdealPFdbkVariant=Disabled  SatFdbkVariant=Disabled  DerivativeFilterVariant=ContFilter  NVariant=InternalParameters  NCopyVariant=Disabled  FilterICVariant=InternalICsFilter  IntegratorICVariant=InternalICs  ExternalResetVariant=Disabled  TRSumVariant=Passthrough  SumFdbkVariant=Disabled  SumVariant=Sum_PID  TsampFilterVariant=InternalTs  TsampNgainVariant=Passthrough  TsampIntegralVariant=Passthrough  ExternalSaturationOutDataTypeStr=Inherit: Same as second input
  PID Controller7 : slpidlib/PID Controller  Controller=PID  Form=Parallel  TimeDomain=Continuous-time  UseExternalTs=off  SampleTime=-1  IntegratorMethod=Forward Euler  FilterMethod=Forward Euler  ControllerParametersSource=internal  P=0.013462751880451  I=6.03710934436948e-04  UseKiTs=off  D=0.667051880736134  N=87.8445721553921  UseFilter=on  TunerSelectOption=Transfer Function Based (PID Tuner App)  InitialConditionSource=internal  InitialConditionForIntegrator=0  InitialConditionForFilter=0  DifferentiatorICPrevScaledInput=0  ExternalReset=none  TrackingMode=off  Kt=1  LimitOutput=on  SatLimitsSource=internal  UpperSaturationLimit=0.52  LowerSaturationLimit=-0.52  LinearizeAsGain=on  AntiWindupMode=none  Kb=1  LimitIntegrator=off  UpperIntegratorSaturationLimit=inf  LowerIntegratorSaturationLimit=-inf  POutMin=[]  POutMax=[]  IOutMin=[]  IOutMax=[]  DOutMin=[]  DOutMax=[]  NOutMin=[]  NOutMax=[]  SumOutMin=[]  SumOutMax=[]  SaturationOutMin=[]  SaturationOutMax=[]  PParamMin=[]  PParamMax=[]  IParamMin=[]  IParamMax=[]  DParamMin=[]  DParamMax=[]  NParamMin=[]  NParamMax=[]  KbParamMin=[]  KbParamMax=[]  KtParamMin=[]  KtParamMax=[]  KbOutMin=[]  KbOutMax=[]  KtOutMin=[]  KtOutMax=[]  IntegratorOutMin=[]  IntegratorOutMax=[]  FilterOutMin=[]  FilterOutMax=[]  SumI1OutMin=[]  SumI1OutMax=[]  SumI2OutMin=[]  SumI2OutMax=[]  SumI3OutMin=[]  SumI3OutMax=[]  SumI4OutMin=[]  SumI4OutMax=[]  SumDOutMin=[]  SumDOutMax=[]  DifferentiatorOutMin=[]  DifferentiatorOutMax=[]  FilterDiffOutCoefMin=[]  FilterDiffOutCoefMax=[]  ReciprocalOutMin=[]  ReciprocalOutMax=[]  SumDenOutMin=[]  SumDenOutMax=[]  SumNumOutMin=[]  SumNumOutMax=[]  DivideOutMin=[]  DivideOutMax=[]  UdiffTsProdOutMin=[]  UdiffTsProdOutMax=[]  NTsProdOutMin=[]  NTsProdOutMax=[]  UintegralTsProdOutMin=[]  UintegralTsProdOutMax=[]  UngainTsProdOutMin=[]  UngainTsProdOutMax=[]  ClampingZeroOutDataTypeStr=Inherit: Inherit via back propagation  ClampingZeroOutMin=[]  ClampingZeroOutMax=[]  FilterDenConstantOutDataTypeStr=Inherit: Inherit via back propagation  FilterDenConstantOutMin=[]  FilterDenConstantOutMax=[]  PCopyOutDataTypeStr=Inherit: Inherit via back propagation  PCopyOutMin=[]  PCopyOutMax=[]  NCopyOutDataTypeStr=Inherit: Inherit via back propagation  NCopyOutMin=[]  NCopyOutMax=[]  IntegratorContinuousStateAttributes=''  IntegratorStateMustResolveToSignalObject=off  IntegratorRTWStateStorageClass=Auto  FilterContinuousStateAttributes=''  FilterStateMustResolveToSignalObject=off  FilterRTWStateStorageClass=Auto  ParallelPVariant=InternalParameters  IdealPVariant=Disabled  IVariant=InternalParameters  DVariant=InternalParameters  IntegratorVariant=Continuous  SatVariant=Enabled  AWVariant=Passthrough  PCopyVariant=Disabled  TRVariant=Disabled  FdbkBlocksVariant=Forward  IdealPFdbkVariant=Disabled  SatFdbkVariant=Disabled  DerivativeFilterVariant=ContFilter  NVariant=InternalParameters  NCopyVariant=Disabled  FilterICVariant=InternalICsFilter  IntegratorICVariant=InternalICs  ExternalResetVariant=Disabled  TRSumVariant=Passthrough  SumFdbkVariant=Disabled  SumVariant=Sum_PID  TsampFilterVariant=InternalTs  TsampNgainVariant=Passthrough  TsampIntegralVariant=Passthrough  ExternalSaturationOutDataTypeStr=Inherit: Same as second input
  Step demand for testing2 : Subsystem
  Subtract2 : Sum  Inputs=|+-
  dA : Outport
  dR : Outport  Port=2
  wires:
  Subtract2/1 -> PID Controller2/1, PID Controller7/1
  Course Angle/1 -> Step demand for testing2/1(Va), Subtract2/1
  PID Controller7/1 -> dA/1
  PID Controller2/1 -> dR/1
  In2/1 -> Subtract2/2

== system Cruise_Model_V16/Trim Solver and Actuation/Controller/PID_GBDP_withThrust/Get angular properties ==
  alpha : Inport
  In2 : Inport  Port=2
  Bus Selector : BusSelector  OutputSignals=EA,uvw,pqr
  Demux1 : Demux  Outputs=3
  Demux2 : Demux  Outputs=3
  Demux3 : Demux  Outputs=3
  Sum : Sum  Inputs=-+|
  Flight Trajectory (gamma) : Outport
  Pitch rate (q) : Outport  Port=2
  ub : Outport  Port=3
  Roll Rate (p) : Outport  Port=4
  Yaw Rate (r) : Outport  Port=5
  Course Angle : Outport  Port=6
  wires:
  alpha/1 -> Sum/1
  Demux2/2 -> Sum/2  "EA"
  Bus Selector/3 -> Demux3/1  "<pqr>"
  Sum/1 -> Flight Trajectory (gamma)/1  "Flight Trajectory (gamma)"
  Bus Selector/1 -> Demux2/1  "<EA>"
  In2/1 -> Bus Selector/1
  Demux3/2 -> Pitch rate (q)/1  "Pitch rate (q)"
  Bus Selector/2 -> Demux1/1  "<uvw>"
  Demux1/1 -> ub/1
  Demux3/1 -> Roll Rate (p)/1
  Demux2/3 -> Course Angle/1
  Demux3/3 -> Yaw Rate (r)/1

== system Cruise_Model_V16/Trim Solver and Actuation/Controller/PID_GBDP_withThrust/Subsystem ==
  note: Airspeed Control Path
  Va : Inport
  Demand : Inport  Port=2
  PID Controller1 : slpidlib/PID Controller  Controller=PID  Form=Parallel  TimeDomain=Continuous-time  UseExternalTs=off  SampleTime=-1  IntegratorMethod=Forward Euler  FilterMethod=Forward Euler  ControllerParametersSource=internal  P=-124.171962714531  I=-8.86566238209981  UseKiTs=off  D=35.5117343437496  UseExternalDerivativeSource=off  N=0.73276571825447  UseFilter=on  TunerSelectOption=Transfer Function Based (PID Tuner App)  InitialConditionSource=internal  InitialConditionForIntegrator=0  InitialConditionForFilter=1  DifferentiatorICPrevScaledInput=0  ExternalReset=none  TrackingMode=off  Kt=1  LimitOutput=on  SatLimitsSource=internal  UpperSaturationLimit=300  LowerSaturationLimit=0  LinearizeAsGain=on  AntiWindupMode=clamping  Kb=1  LimitIntegrator=off  UpperIntegratorSaturationLimit=inf  LowerIntegratorSaturationLimit=-inf  POutMin=[]  POutMax=[]  IOutMin=[]  IOutMax=[]  DOutMin=[]  DOutMax=[]  NOutMin=[]  NOutMax=[]  SumOutMin=[]  SumOutMax=[]  SaturationOutMin=[]  SaturationOutMax=[]  PParamMin=[]  PParamMax=[]  IParamMin=[]  IParamMax=[]  DParamMin=[]  DParamMax=[]  NParamMin=[]  NParamMax=[]  KbParamMin=[]  KbParamMax=[]  KtParamMin=[]  KtParamMax=[]  KbOutMin=[]  KbOutMax=[]  KtOutMin=[]  KtOutMax=[]  IntegratorOutMin=[]  IntegratorOutMax=[]  FilterOutMin=[]  FilterOutMax=[]  SumI1OutMin=[]  SumI1OutMax=[]  SumI2OutMin=[]  SumI2OutMax=[]  SumI3OutMin=[]  SumI3OutMax=[]  SumI4OutMin=[]  SumI4OutMax=[]  SumDOutMin=[]  SumDOutMax=[]  DifferentiatorOutMin=[]  DifferentiatorOutMax=[]  FilterDiffOutCoefMin=[]  FilterDiffOutCoefMax=[]  ReciprocalOutMin=[]  ReciprocalOutMax=[]  SumDenOutMin=[]  SumDenOutMax=[]  SumNumOutMin=[]  SumNumOutMax=[]  DivideOutMin=[]  DivideOutMax=[]  UdiffTsProdOutMin=[]  UdiffTsProdOutMax=[]  NTsProdOutMin=[]  NTsProdOutMax=[]  UintegralTsProdOutMin=[]  UintegralTsProdOutMax=[]  UngainTsProdOutMin=[]  UngainTsProdOutMax=[]  ClampingZeroOutDataTypeStr=Inherit: Inherit via back propagation  ClampingZeroOutMin=[]  ClampingZeroOutMax=[]  FilterDenConstantOutDataTypeStr=Inherit: Inherit via back propagation  FilterDenConstantOutMin=[]  FilterDenConstantOutMax=[]  PCopyOutDataTypeStr=Inherit: Inherit via back propagation  PCopyOutMin=[]  PCopyOutMax=[]  NCopyOutDataTypeStr=Inherit: Inherit via back propagation  NCopyOutMin=[]  NCopyOutMax=[]  IntegratorContinuousStateAttributes=''  IntegratorStateMustResolveToSignalObject=off  IntegratorRTWStateStorageClass=Auto  FilterContinuousStateAttributes=''  FilterStateMustResolveToSignalObject=off  FilterRTWStateStorageClass=Auto  ParallelPVariant=InternalParameters  IdealPVariant=Disabled  IVariant=InternalParameters  DVariant=InternalParameters  IntegratorVariant=Continuous  SatVariant=Enabled  AWVariant=ContClampingParallel  PCopyVariant=Disabled  TRVariant=Disabled  FdbkBlocksVariant=Forward  IdealPFdbkVariant=Disabled  SatFdbkVariant=Disabled  DerivativeFilterVariant=ContFilter  NVariant=InternalParameters  NCopyVariant=Disabled  FilterICVariant=InternalICsFilter  IntegratorICVariant=InternalICs  ExternalResetVariant=Disabled  TRSumVariant=Passthrough  SumFdbkVariant=Disabled  SumVariant=Sum_PID  TsampFilterVariant=InternalTs  TsampNgainVariant=Passthrough  TsampIntegralVariant=Disabled_SignalSpec  ExternalSaturationOutDataTypeStr=Inherit: Same as second input  DerivativeSourceVariant=ErrorSignal
  Step demand for testing1 : Subsystem
  Subtract5 : Sum  Inputs=|+-
  dT : Outport
  wires:
  PID Controller1/1 -> dT/1
  Subtract5/1 -> PID Controller1/1
  Va/1 -> Subtract5/1, Step demand for testing1/1(Va)
  Demand/1 -> Subtract5/2
  Step demand for testing1/1(Out1) -> ?

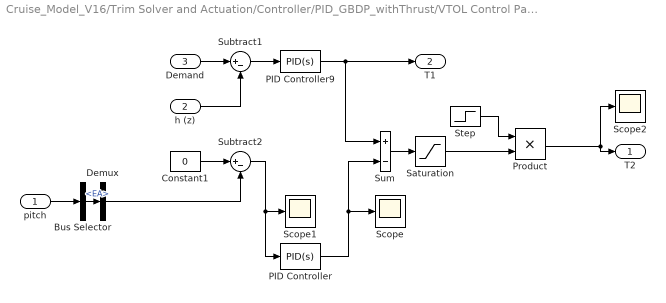
== system Cruise_Model_V16/Trim Solver and Actuation/Controller/PID_GBDP_withThrust/VTOL Control Path ==
  pitch : Inport
  h (z) : Inport  Port=2
  Demand : Inport  Port=3
  Bus Selector : BusSelector  OutputSignals=EA
  Constant1 : Constant  Value=0
  Demux : Demux  Outputs=3
  PID Controller : slpidlib/PID Controller  Controller=PID  Form=Parallel  TimeDomain=Continuous-time  UseExternalTs=off  SampleTime=-1  IntegratorMethod=Forward Euler  FilterMethod=Forward Euler  ControllerParametersSource=internal  P=2347  I=2604  UseKiTs=off  D=519  N=129  UseFilter=on  TunerSelectOption=Transfer Function Based (PID Tuner App)  InitialConditionSource=internal  InitialConditionForIntegrator=0  InitialConditionForFilter=0  DifferentiatorICPrevScaledInput=0  ExternalReset=none  TrackingMode=off  Kt=1  LimitOutput=on  SatLimitsSource=internal  UpperSaturationLimit=800  LowerSaturationLimit=-800  LinearizeAsGain=on  AntiWindupMode=clamping  Kb=1  LimitIntegrator=off  UpperIntegratorSaturationLimit=inf  LowerIntegratorSaturationLimit=-inf  POutMin=[]  POutMax=[]  IOutMin=[]  IOutMax=[]  DOutMin=[]  DOutMax=[]  NOutMin=[]  NOutMax=[]  SumOutMin=[]  SumOutMax=[]  SaturationOutMin=[]  SaturationOutMax=[]  PParamMin=[]  PParamMax=[]  IParamMin=[]  IParamMax=[]  DParamMin=[]  DParamMax=[]  NParamMin=[]  NParamMax=[]  KbParamMin=[]  KbParamMax=[]  KtParamMin=[]  KtParamMax=[]  KbOutMin=[]  KbOutMax=[]  KtOutMin=[]  KtOutMax=[]  IntegratorOutMin=[]  IntegratorOutMax=[]  FilterOutMin=[]  FilterOutMax=[]  SumI1OutMin=[]  SumI1OutMax=[]  SumI2OutMin=[]  SumI2OutMax=[]  SumI3OutMin=[]  SumI3OutMax=[]  SumI4OutMin=[]  SumI4OutMax=[]  SumDOutMin=[]  SumDOutMax=[]  DifferentiatorOutMin=[]  DifferentiatorOutMax=[]  FilterDiffOutCoefMin=[]  FilterDiffOutCoefMax=[]  ReciprocalOutMin=[]  ReciprocalOutMax=[]  SumDenOutMin=[]  SumDenOutMax=[]  SumNumOutMin=[]  SumNumOutMax=[]  DivideOutMin=[]  DivideOutMax=[]  UdiffTsProdOutMin=[]  UdiffTsProdOutMax=[]  NTsProdOutMin=[]  NTsProdOutMax=[]  UintegralTsProdOutMin=[]  UintegralTsProdOutMax=[]  UngainTsProdOutMin=[]  UngainTsProdOutMax=[]  ClampingZeroOutDataTypeStr=Inherit: Inherit via back propagation  ClampingZeroOutMin=[]  ClampingZeroOutMax=[]  FilterDenConstantOutDataTypeStr=Inherit: Inherit via back propagation  FilterDenConstantOutMin=[]  FilterDenConstantOutMax=[]  PCopyOutDataTypeStr=Inherit: Inherit via back propagation  PCopyOutMin=[]  PCopyOutMax=[]  NCopyOutDataTypeStr=Inherit: Inherit via back propagation  NCopyOutMin=[]  NCopyOutMax=[]  IntegratorContinuousStateAttributes=''  IntegratorStateMustResolveToSignalObject=off  IntegratorRTWStateStorageClass=Auto  FilterContinuousStateAttributes=''  FilterStateMustResolveToSignalObject=off  FilterRTWStateStorageClass=Auto  ParallelPVariant=InternalParameters  IdealPVariant=Disabled  IVariant=InternalParameters  DVariant=InternalParameters  IntegratorVariant=Continuous  SatVariant=Enabled  AWVariant=ContClampingParallel  PCopyVariant=Disabled  TRVariant=Disabled  FdbkBlocksVariant=Forward  IdealPFdbkVariant=Disabled  SatFdbkVariant=Disabled  DerivativeFilterVariant=ContFilter  NVariant=InternalParameters  NCopyVariant=Disabled  FilterICVariant=InternalICsFilter  IntegratorICVariant=InternalICs  ExternalResetVariant=Disabled  TRSumVariant=Passthrough  SumFdbkVariant=Disabled  SumVariant=Sum_PID  TsampFilterVariant=InternalTs  TsampNgainVariant=Passthrough  TsampIntegralVariant=Passthrough  ExternalSaturationOutDataTypeStr=Inherit: Same as second input
  PID Controller9 : slpidlib/PID Controller  Controller=PID  Form=Parallel  TimeDomain=Continuous-time  UseExternalTs=off  SampleTime=-1  IntegratorMethod=Forward Euler  FilterMethod=Forward Euler  ControllerParametersSource=internal  P=-174.901958260333  I=-41.0371926298995  UseKiTs=off  D=-183.043785953636  N=27.3346026399604  UseFilter=on  TunerSelectOption=Transfer Function Based (PID Tuner App)  InitialConditionSource=internal  InitialConditionForIntegrator=0  InitialConditionForFilter=0  DifferentiatorICPrevScaledInput=0  ExternalReset=none  TrackingMode=off  Kt=1  LimitOutput=on  SatLimitsSource=internal  UpperSaturationLimit=2000  LowerSaturationLimit=0  LinearizeAsGain=off  AntiWindupMode=clamping  Kb=1  LimitIntegrator=off  UpperIntegratorSaturationLimit=inf  LowerIntegratorSaturationLimit=-inf  POutMin=[]  POutMax=[]  IOutMin=[]  IOutMax=[]  DOutMin=[]  DOutMax=[]  NOutMin=[]  NOutMax=[]  SumOutMin=[]  SumOutMax=[]  SaturationOutMin=[]  SaturationOutMax=[]  PParamMin=[]  PParamMax=[]  IParamMin=[]  IParamMax=[]  DParamMin=[]  DParamMax=[]  NParamMin=[]  NParamMax=[]  KbParamMin=[]  KbParamMax=[]  KtParamMin=[]  KtParamMax=[]  KbOutMin=[]  KbOutMax=[]  KtOutMin=[]  KtOutMax=[]  IntegratorOutMin=[]  IntegratorOutMax=[]  FilterOutMin=[]  FilterOutMax=[]  SumI1OutMin=[]  SumI1OutMax=[]  SumI2OutMin=[]  SumI2OutMax=[]  SumI3OutMin=[]  SumI3OutMax=[]  SumI4OutMin=[]  SumI4OutMax=[]  SumDOutMin=[]  SumDOutMax=[]  DifferentiatorOutMin=[]  DifferentiatorOutMax=[]  FilterDiffOutCoefMin=[]  FilterDiffOutCoefMax=[]  ReciprocalOutMin=[]  ReciprocalOutMax=[]  SumDenOutMin=[]  SumDenOutMax=[]  SumNumOutMin=[]  SumNumOutMax=[]  DivideOutMin=[]  DivideOutMax=[]  UdiffTsProdOutMin=[]  UdiffTsProdOutMax=[]  NTsProdOutMin=[]  NTsProdOutMax=[]  UintegralTsProdOutMin=[]  UintegralTsProdOutMax=[]  UngainTsProdOutMin=[]  UngainTsProdOutMax=[]  ClampingZeroOutDataTypeStr=Inherit: Inherit via back propagation  ClampingZeroOutMin=[]  ClampingZeroOutMax=[]  FilterDenConstantOutDataTypeStr=Inherit: Inherit via back propagation  FilterDenConstantOutMin=[]  FilterDenConstantOutMax=[]  PCopyOutDataTypeStr=Inherit: Inherit via back propagation  PCopyOutMin=[]  PCopyOutMax=[]  NCopyOutDataTypeStr=Inherit: Inherit via back propagation  NCopyOutMin=[]  NCopyOutMax=[]  IntegratorContinuousStateAttributes=''  IntegratorStateMustResolveToSignalObject=off  IntegratorRTWStateStorageClass=Auto  FilterContinuousStateAttributes=''  FilterStateMustResolveToSignalObject=off  FilterRTWStateStorageClass=Auto  ParallelPVariant=InternalParameters  IdealPVariant=Disabled  IVariant=InternalParameters  DVariant=InternalParameters  IntegratorVariant=Continuous  SatVariant=Enabled  AWVariant=ContClampingParallel  PCopyVariant=Disabled  TRVariant=Disabled  FdbkBlocksVariant=Forward  IdealPFdbkVariant=Disabled  SatFdbkVariant=Disabled  DerivativeFilterVariant=ContFilter  NVariant=InternalParameters  NCopyVariant=Disabled  FilterICVariant=InternalICsFilter  IntegratorICVariant=InternalICs  ExternalResetVariant=Disabled  TRSumVariant=Passthrough  SumFdbkVariant=Disabled  SumVariant=Sum_PID  TsampFilterVariant=InternalTs  TsampNgainVariant=Passthrough  TsampIntegralVariant=Passthrough  ExternalSaturationOutDataTypeStr=Inherit: Same as second input
  Product : Product
  Saturation : Saturate  UpperLimit=9000  LowerLimit=0
  Scope : Scope
  Scope1 : Scope
  Scope2 : Scope
  Step : Step  Time=max(mission.trans.t)  Before=1  After=0  SampleTime=0
  Subtract1 : Sum  Inputs=|+-
  Subtract2 : Sum  Inputs=|+-
  Sum : Sum  Inputs=+-
  T2 : Outport
  T1 : Outport  Port=2
  wires:
  Demand/1 -> Subtract1/1
  h (z)/1 -> Subtract1/2
  Subtract1/1 -> PID Controller9/1
  Constant1/1 -> Subtract2/1
  pitch/1 -> Bus Selector/1
  Subtract2/1 -> PID Controller/1, Scope1/1
  PID Controller9/1 -> Sum/1, T1/1
  Sum/1 -> Saturation/1
  PID Controller/1 -> Sum/2, Scope/1
  Bus Selector/1 -> Demux/1  "<EA>"
  Demux/2 -> Subtract2/2
  Product/1 -> T2/1, Scope2/1
  Saturation/1 -> Product/2
  Step/1 -> Product/1
